simulink model "top_model_24a"  (R2024a)
settings: Solver=VariableStepAuto  StartTime=0.0  StopTime=90  RelTol=1e-3  EnableMultiTasking=on
values from neighbouring files (symbols this model uses):
  target = waypoints(idx, :)'    [waypointFollower - Copy.m]    (also in waypointFollower.m)
undefined symbols (not defined in the file or in its folder): controller, gray, vehicle, X, Y, Z
libraries: sm_lib x13, nesl_utility x6, simulink x5, slpidlib x2, robotmobilelib x1
(part 1 of 2)
settings Model: Creator=The MathWorks, Inc.  LastModifiedBy=s1706516
settings SolverCC: AlgebraicLoopSolver=TrustRegion
settings DataIOCC: LimitDataPoints=on  ReturnWorkspaceOutputs=off
settings OptimizationCC: LifeSpan=inf
settings DebuggingCC: UnconnectedInputMsg=warning  UnconnectedOutputMsg=warning  UnconnectedLineMsg=warning  AllowSymbolicDim=off  SFUnexpectedBacktrackingDiag=warning  SFNoUnconditionalDefaultTransitionDiag=warning  SFExecutionAtInitializationDiag=none  ArithmeticOperatorsInVariantConditions=warning
settings ModelReferenceCC: EnableRefExpFcnMdlSchedulingChecks=on  PropagateSignalLabelsOutOfModel=off
settings SFSimCC: SimUseLocalCustomCode=off  CustomCodeUndefinedFunction=UseInterfaceOnly
settings RTWCC: RTWUseLocalCustomCode=off  GPUComputeCapability=3.5
settings CodeAppCC: StateflowObjectComments=on
settings GRTTargetCC: TargetLangStandard=C89/C90 (ANSI)
settings ConfigComp: CovMetricSettings=dw  CovSaveCumulativeToWorkspaceVar=on  CovSaveSingleToWorkspaceVar=on  CovExternalEMLEnable=off
settings ExplorerConfigSet: InternalSimMechanicsExplorerSettings="<ExplorerConfiguration><canonicalview>default</canonicalview><AnimationSetting><BasePlaybackSpeed>1.0</BasePlaybackSpeed><PlaybackSpeedFactor>1.0</PlaybackSpeedFactor></AnimationSetting><TilePanel><TileInfo><Tiles Columns=\"1\" Count=\"1\" Rows=\"1\"><Column Weight=\"1\"/><Row Weight=\"1\"/><Tile Height=\"1\" Width=\"1\" X=\"0\" Y=\"0\"/></Tiles></TileInfo><SceneInfo><SceneViewer><BGColor><R>0.60000002384185791</R><G>0.60000002384185791</G><B>0.60000002384185791</B></BGColor><Camera><DoPerspective>off</DoPerspective><Position><X>8.17861551168531875</X><Y>-8.17861559442319219</Y><Z>8.17861528352223388</Z></Position><Center><X>9.49663426935732896e-08</X><Y>-1.77704216256942048e-07</Y><Z>-1.33196743078566375e-07</Z></Center><Up><X>-0.408248290463863073</X><Y>0.408248290463863073</Y><Z>0.816496580927726145</Z></Up><ViewLimDist>1</ViewLimDist><YLim>8.40991459846496525</YLim><XLim>17.077552386237727</XLim></Camera></SceneViewer></SceneInfo></TilePanel><MechEditorPanel><Cameras/><GfxPanelCameraMap/><VideoCreator><PlaybackSpeedRatio>1.0</PlaybackSpeedRatio><FrameRate>30</FrameRate><VideoFormat>Motion JPEG AVI</VideoFormat><FrameSize>auto</FrameSize></VideoCreator></MechEditorPanel></ExplorerConfiguration>"

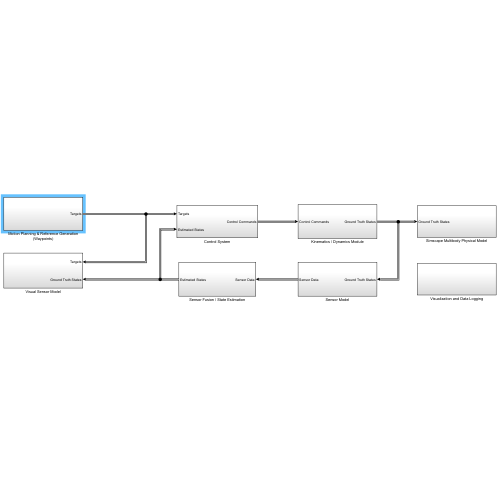
[thumbnail: Simulink's stored preview of the top-level diagram]
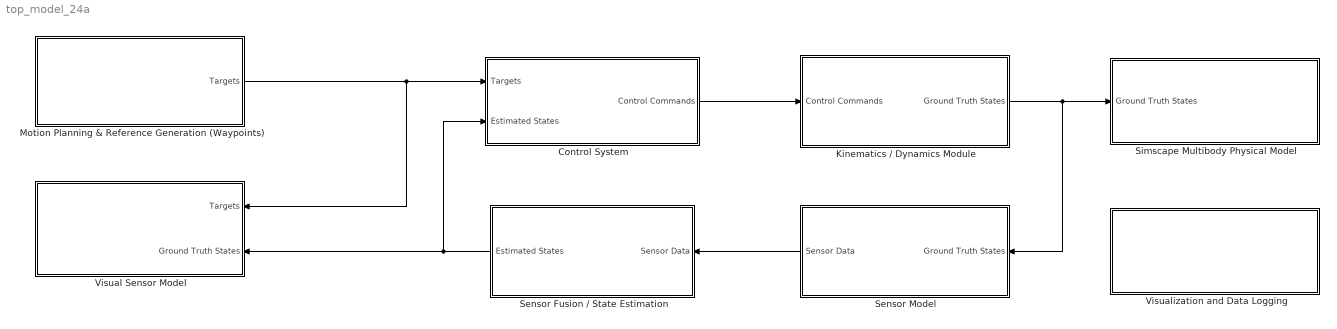
== system top_model_24a ==
  Control System : Subsystem
  Kinematics / Dynamics Module : Subsystem
  Motion Planning & Reference Generation (Waypoints) : Subsystem
  Sensor Fusion / State Estimation : Subsystem
  Sensor Model : Subsystem
  Simscape Multibody Physical Model : Subsystem
  Visual Sensor Model : Subsystem
  Visualization and Data Logging : Subsystem
  wires:
  Sensor Model/1(Sensor Data) -> Sensor Fusion / State Estimation/1(Sensor Data)
  Sensor Fusion / State Estimation/1(Estimated States) -> Visual Sensor Model/2(Ground Truth States), Control System/2(Estimated States)
  Control System/1(Control Commands) -> Kinematics / Dynamics Module/1(Control Commands)
  Kinematics / Dynamics Module/1(Ground Truth States) -> Sensor Model/1(Ground Truth States), Simscape Multibody Physical Model/1(Ground Truth States)
  Motion Planning & Reference Generation (Waypoints)/1(Targets) -> Visual Sensor Model/1(Targets), Control System/1(Targets)

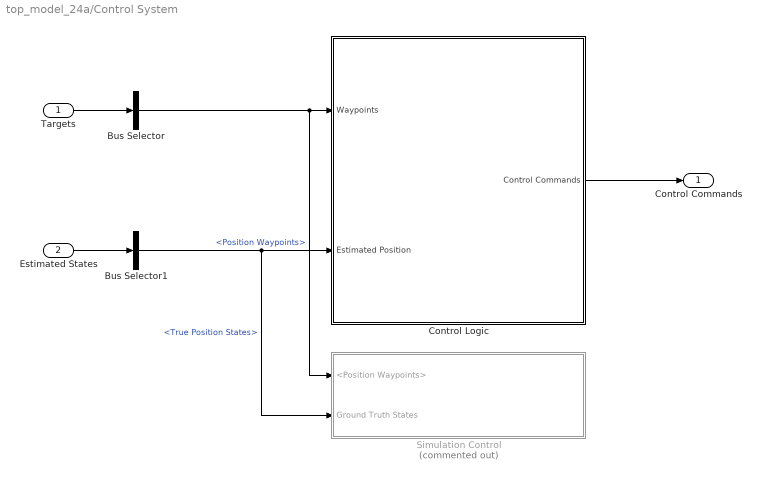
== system top_model_24a/Control System ==
  Targets : Inport
  Estimated States : Inport  Port=2
  Bus Selector : BusSelector  OutputSignals=Position Waypoints
  Bus Selector1 : BusSelector  OutputSignals=True Position States
  Control Logic : Subsystem
  Simulation Control : Subsystem  Commented=on
  Control Commands : Outport
  wires:
  Estimated States/1 -> Bus Selector1/1
  Bus Selector/1 -> Simulation Control/1(<Position Waypoints>), Control Logic/1(Waypoints)  "<Position Waypoints>"
  Targets/1 -> Bus Selector/1
  Control Logic/1(Control Commands) -> Control Commands/1
  Bus Selector1/1 -> Simulation Control/2(Ground Truth States), Control Logic/2(Estimated Position)  "<True Position States>"

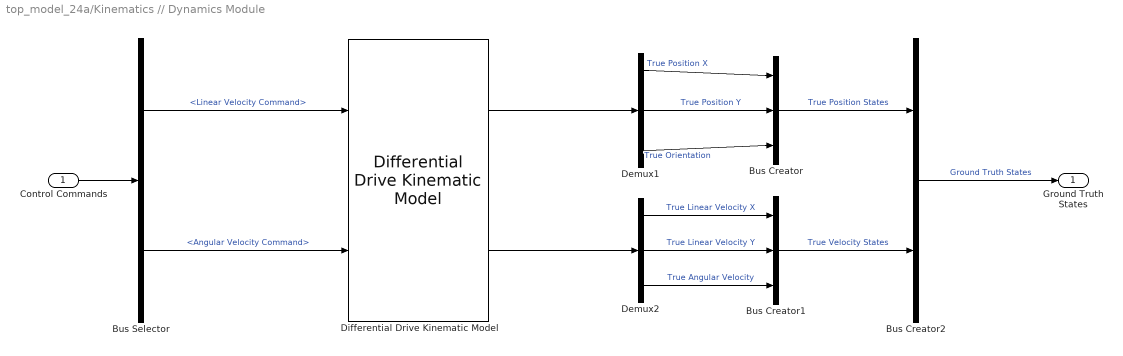
== system top_model_24a/Kinematics // Dynamics Module ==
  Control Commands : Inport
  Bus Creator : BusCreator  Inputs=3
  Bus Creator1 : BusCreator  Inputs=3
  Bus Creator2 : BusCreator  Inputs=2
  Bus Selector : BusSelector  OutputSignals=Linear Velocity Command,Angular Velocity Command
  Demux1 : Demux  Outputs=3
  Demux2 : Demux  Outputs=3
  Differential Drive Kinematic Model : robotmobilelib/Differential Drive Kinematic Model  VehicleInputs=Vehicle Speed & Heading Angular Velocity  WheelRadius=vehicle.wheel.radius  WheelSpeedRange=[-inf inf]  TrackWidth=vehicle.wheel.width  InitialState=init.vehicle.state  SimulateUsing=Interpreted execution
  Ground Truth States : Outport
  wires:
  Bus Selector/1 -> Differential Drive Kinematic Model/1  "<Linear Velocity Command>"
  Bus Selector/2 -> Differential Drive Kinematic Model/2  "<Angular Velocity Command>"
  Control Commands/1 -> Bus Selector/1
  Differential Drive Kinematic Model/1 -> Demux1/1
  Demux1/2 -> Bus Creator/2  "True Position Y"
  Demux1/1 -> Bus Creator/1  "True Position X"
  Demux1/3 -> Bus Creator/3  "True Orientation"
  Differential Drive Kinematic Model/2 -> Demux2/1
  Demux2/1 -> Bus Creator1/1  "True Linear Velocity X"
  Demux2/3 -> Bus Creator1/3  "True Angular Velocity"
  Demux2/2 -> Bus Creator1/2  "True Linear Velocity Y"
  Bus Creator/1 -> Bus Creator2/1  "True Position States"
  Bus Creator1/1 -> Bus Creator2/2  "True Velocity States"
  Bus Creator2/1 -> Ground Truth States/1  "Ground Truth States"

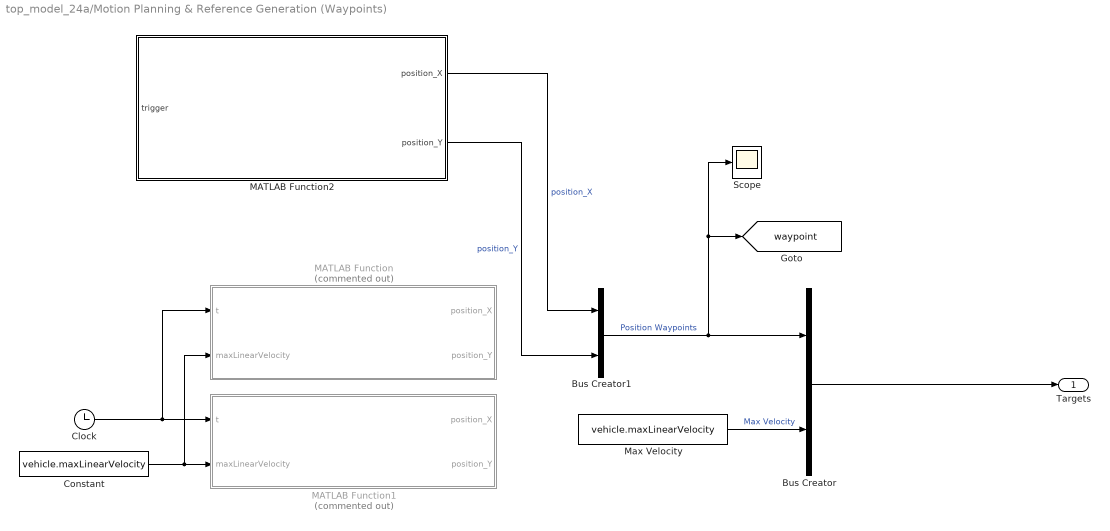
== system top_model_24a/Motion Planning & Reference Generation (Waypoints) ==
  Bus Creator : BusCreator  Inputs=2
  Bus Creator1 : BusCreator  Inputs=2
  Clock : Clock
  Constant : Constant  Value=vehicle.maxLinearVelocity
  MATLAB Function : MATLAB Function  Commented=on  TreatAsAtomicUnit=on
  MATLAB Function1 : MATLAB Function  Commented=on  TreatAsAtomicUnit=on
  MATLAB Function2 : MATLAB Function  TreatAsAtomicUnit=on
  Max Velocity : Constant  Value=vehicle.maxLinearVelocity
  Scope : Scope
  Targets : Outport
  tag scope: waypoint=global
  wires:
  Max Velocity/1 -> Bus Creator/2  "Max Velocity"
  Bus Creator/1 -> Targets/1
  Bus Creator1/1 -> Bus Creator/1, [waypoint], Scope/1  "Position Waypoints"
  Constant/1 -> MATLAB Function/2(maxLinearVelocity), MATLAB Function1/2(maxLinearVelocity)
  Clock/1 -> MATLAB Function/1(t), MATLAB Function1/1(t)
  MATLAB Function2/1(position_X) -> Bus Creator1/1  "position_X"
  MATLAB Function2/2(position_Y) -> Bus Creator1/2  "position_Y"

== system top_model_24a/Sensor Fusion // State Estimation ==
  Sensor Data : Inport
  Bus Creator : BusCreator  Inputs=2
  Bus Selector : BusSelector  OutputSignals=True Position States,True Velocity States
  Sensor Fusion : Subsystem
  Estimated States : Outport
  wires:
  Sensor Data/1 -> Bus Selector/1  "Sensor Data"
  Bus Creator/1 -> Estimated States/1  "Estimated States"
  Bus Selector/1 -> Sensor Fusion/1(In1)  "<True Position States>"
  Bus Selector/2 -> Sensor Fusion/2(In2)  "<True Velocity States>"
  Sensor Fusion/1(Out1) -> Bus Creator/1
  Sensor Fusion/2(Out2) -> Bus Creator/2

== system top_model_24a/Sensor Model ==
  Ground Truth States : Inport
  Sensors : Subsystem
  Switch : simulink/Signal Routing/Manual Variant Source  NumChoices=2  LabelModeActiveChoice=V_1
  True Feedthrough : Subsystem
  Sensor Data : Outport
  wires:
  Switch/1 -> Sensor Data/1
  Ground Truth States/1 -> True Feedthrough/1(Ground Truth States), Sensors/1(Ground Truth States)
  Sensors/1(Simulated Raw Sensor Data) -> Switch/1  "Sensor Data"
  True Feedthrough/1(True Feedthrough Sensor Data) -> Switch/2  "Sensor Data"

== system top_model_24a/Simscape Multibody Physical Model ==
  Ground Truth States : Inport
  Bus Selector : BusSelector  OutputSignals=True Position States
  Simscape Model : Subsystem
  wires:
  Ground Truth States/1 -> Bus Selector/1
  Bus Selector/1 -> Simscape Model/1(True Position States)  "<True Position States>"

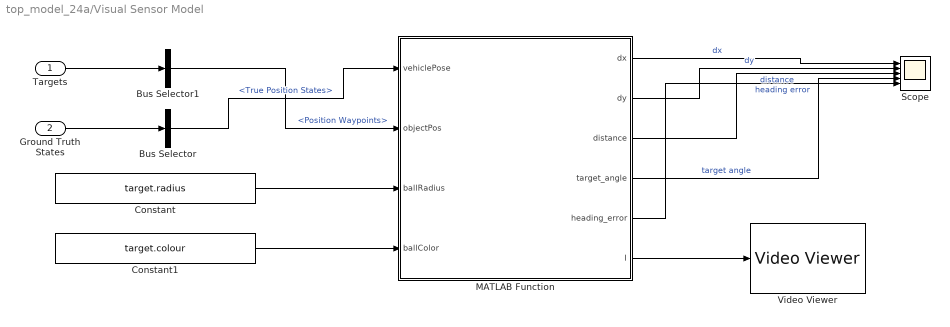
== system top_model_24a/Visual Sensor Model ==
  Targets : Inport
  Ground Truth States : Inport  Port=2
  Bus Selector : BusSelector  OutputSignals=True Position States
  Bus Selector1 : BusSelector  OutputSignals=Position Waypoints
  Constant : Constant  Value=target.radius
  Constant1 : Constant  Value=target.colour
  MATLAB Function : MATLAB Function  TreatAsAtomicUnit=on
  Scope : Scope  NumInputPorts=5
  Video Viewer : VideoViewer  colormapValue=gray(256)  FigPos=[830 505 439 384]
  wires:
  Ground Truth States/1 -> Bus Selector/1
  Bus Selector/1 -> MATLAB Function/1(vehiclePose)  "<True Position States>"
  Targets/1 -> Bus Selector1/1
  Bus Selector1/1 -> MATLAB Function/2(objectPos)  "<Position Waypoints>"
  MATLAB Function/6(I) -> Video Viewer/1
  Constant/1 -> MATLAB Function/3(ballRadius)
  Constant1/1 -> MATLAB Function/4(ballColor)
  MATLAB Function/1(dx) -> Scope/1  "dx"
  MATLAB Function/2(dy) -> Scope/2  "dy"
  MATLAB Function/4(target_angle) -> Scope/4  "target angle"
  MATLAB Function/5(heading_error) -> Scope/5  "heading error"
  MATLAB Function/3(distance) -> Scope/3  "distance"

== system top_model_24a/Visualization and Data Logging ==

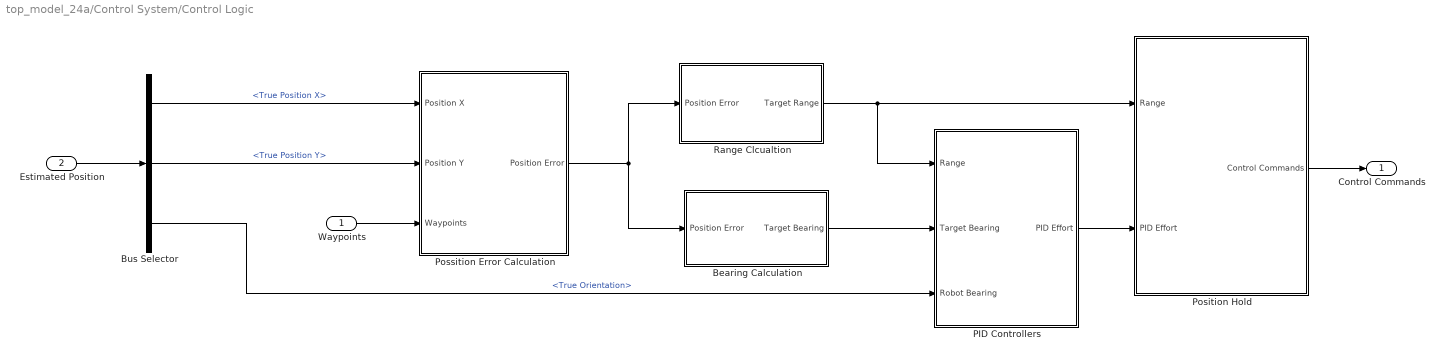
== system top_model_24a/Control System/Control Logic ==
  Waypoints : Inport
  Estimated Position : Inport  Port=2
  Bearing Calculation : Subsystem
  Bus Selector : BusSelector  OutputSignals=True Position X,True Position Y,True Orientation
  PID Controllers : Subsystem
  Position Hold : Subsystem
  Possition Error Calculation : Subsystem
  Range Clcualtion : Subsystem
  Control Commands : Outport
  wires:
  Waypoints/1 -> Possition Error Calculation/3(Waypoints)
  Estimated Position/1 -> Bus Selector/1
  Bus Selector/3 -> PID Controllers/3(Robot Bearing)  "<True Orientation>"
  Position Hold/1(Control Commands) -> Control Commands/1
  Bearing Calculation/1(Target Bearing) -> PID Controllers/2(Target Bearing)
  Possition Error Calculation/1(Position Error) -> Range Clcualtion/1(Position Error), Bearing Calculation/1(Position Error)
  Bus Selector/1 -> Possition Error Calculation/1(Position X)  "<True Position X>"
  Bus Selector/2 -> Possition Error Calculation/2(Position Y)  "<True Position Y>"
  Range Clcualtion/1(Target Range) -> PID Controllers/1(Range), Position Hold/1(Range)
  PID Controllers/1(PID Effort) -> Position Hold/2(PID Effort)

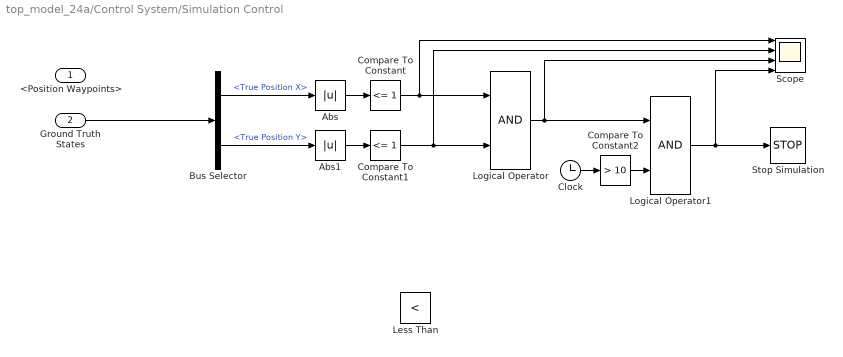
== system top_model_24a/Control System/Simulation Control ==
  <Position Waypoints> : Inport
  Ground Truth States : Inport  Port=2
  Abs : Abs  SaturateOnIntegerOverflow=off
  Abs1 : Abs  SaturateOnIntegerOverflow=off
  Bus Selector : BusSelector  OutputSignals=True Position X,True Position Y
  Clock : Clock
  Compare To Constant : simulink/Logic and Bit Operations/Compare To Constant  relop=<=  const=1  OutDataTypeStr=boolean
  Compare To Constant1 : simulink/Logic and Bit Operations/Compare To Constant  relop=<=  const=1  OutDataTypeStr=boolean
  Compare To Constant2 : simulink/Logic and Bit Operations/Compare To Constant  relop=>  const=10  OutDataTypeStr=boolean
  Less Than : RelationalOperator  Operator=<  OutDataTypeStr=boolean  RndMeth=Simplest  InputSameDT=off
  Logical Operator : Logic  AllPortsSameDT=off  OutDataTypeStr=boolean
  Logical Operator1 : Logic  AllPortsSameDT=off  OutDataTypeStr=boolean
  Scope : Scope  NumInputPorts=4
  Stop Simulation : Stop
  wires:
  Ground Truth States/1 -> Bus Selector/1
  Bus Selector/1 -> Abs/1  "<True Position X>"
  Bus Selector/2 -> Abs1/1  "<True Position Y>"
  Compare To Constant/1 -> Logical Operator/1, Scope/1
  Compare To Constant1/1 -> Logical Operator/2, Scope/2
  Logical Operator/1 -> Logical Operator1/1, Scope/3
  Abs/1 -> Compare To Constant/1
  Abs1/1 -> Compare To Constant1/1
  Compare To Constant2/1 -> Logical Operator1/2
  Clock/1 -> Compare To Constant2/1
  Logical Operator1/1 -> Stop Simulation/1, Scope/4

== system top_model_24a/Sensor Fusion // State Estimation/Sensor Fusion ==
  In1 : Inport
  In2 : Inport  Port=2
  Out1 : Outport
  Out2 : Outport  Port=2
  wires:
  In1/1 -> Out1/1
  In2/1 -> Out2/1

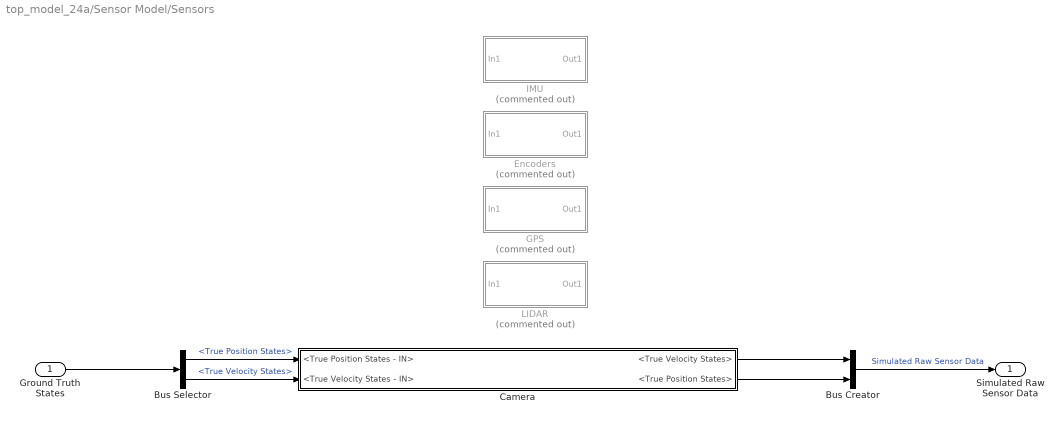
== system top_model_24a/Sensor Model/Sensors ==
  Ground Truth States : Inport
  Bus Creator : BusCreator  Inputs=2
  Bus Selector : BusSelector  OutputSignals=True Position States,True Velocity States
  Camera : Subsystem
  Encoders : Subsystem  Commented=on
  GPS : Subsystem  Commented=on
  IMU : Subsystem  Commented=on
  LIDAR : Subsystem  Commented=on
  Simulated Raw Sensor Data : Outport
  wires:
  Ground Truth States/1 -> Bus Selector/1
  Bus Creator/1 -> Simulated Raw Sensor Data/1  "Simulated Raw Sensor Data"
  Camera/2(<True Position States>) -> Bus Creator/2
  Bus Selector/2 -> Camera/2(<True Velocity States - IN>)  "<True Velocity States>"
  Bus Selector/1 -> Camera/1(<True Position States - IN>)  "<True Position States>"
  Camera/1(<True Velocity States>) -> Bus Creator/1

== system top_model_24a/Sensor Model/True Feedthrough ==
  Ground Truth States : Inport
  Bus Creator : BusCreator  Inputs=2
  Bus Selector : BusSelector  OutputSignals=True Position States,True Velocity States
  True Feedthrough Sensor Data : Outport
  wires:
  Bus Creator/1 -> True Feedthrough Sensor Data/1  "True Feedthrough Sensor Data"
  Ground Truth States/1 -> Bus Selector/1
  Bus Selector/1 -> Bus Creator/1  "<True Position States>"
  Bus Selector/2 -> Bus Creator/2  "<True Velocity States>"

== system top_model_24a/Simscape Multibody Physical Model/Simscape Model ==
  True Position States : Inport
  Vehicle Base : Subsystem
  World and Solver : Subsystem
  wires:
  True Position States/1 -> Vehicle Base/1(True Position States)
  connections:
  World and Solver/RConn1 -- Vehicle Base/LConn1

== system top_model_24a/Control System/Control Logic/Bearing Calculation ==
  Position Error : Inport
  Atan1 : Trigonometry  Operator=atan2
  Demux1 : Demux  Outputs=2
  Target Bearing : Outport
  wires:
  Demux1/2 -> Atan1/1
  Demux1/1 -> Atan1/2
  Atan1/1 -> Target Bearing/1
  Position Error/1 -> Demux1/1

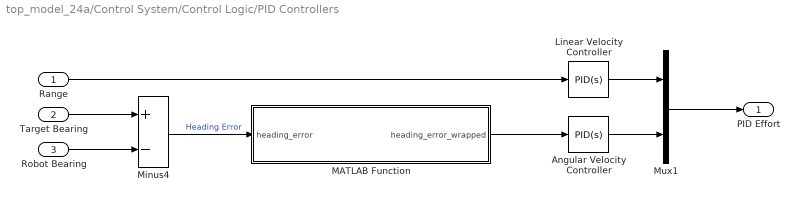
== system top_model_24a/Control System/Control Logic/PID Controllers ==
  Range : Inport
  Target Bearing : Inport  Port=2
  Robot Bearing : Inport  Port=3
  Angular Velocity Controller : slpidlib/PID Controller  Controller=PID  Form=Parallel  TimeDomain=Continuous-time  UseExternalTs=off  SampleTime=-1  IntegratorMethod=Forward Euler  FilterMethod=Forward Euler  ControllerParametersSource=internal  P=1  I=0  UseKiTs=off  D=0.1  UseExternalDerivativeSource=off  N=1  UseFilter=on  TunerSelectOption=Transfer Function Based (PID Tuner App)  InitialConditionSource=internal  InitialConditionForIntegrator=0  InitialConditionForFilter=0  DifferentiatorICPrevScaledInput=0  ExternalReset=none  TrackingMode=off  Kt=1  LimitOutput=off  SatLimitsSource=internal  UpperSaturationLimit=inf  LowerSaturationLimit=-inf  LinearizeAsGain=on  AntiWindupMode=none  Kb=1  LimitIntegrator=off  UpperIntegratorSaturationLimit=inf  LowerIntegratorSaturationLimit=-inf  POutMin=[]  POutMax=[]  IOutMin=[]  IOutMax=[]  DOutMin=[]  DOutMax=[]  NOutMin=[]  NOutMax=[]  SumOutMin=[]  SumOutMax=[]  SaturationOutMin=[]  SaturationOutMax=[]  PParamMin=[]  PParamMax=[]  IParamMin=[]  IParamMax=[]  DParamMin=[]  DParamMax=[]  NParamMin=[]  NParamMax=[]  KbParamMin=[]  KbParamMax=[]  KtParamMin=[]  KtParamMax=[]  KbOutMin=[]  KbOutMax=[]  KtOutMin=[]  KtOutMax=[]  IntegratorOutMin=[]  IntegratorOutMax=[]  FilterOutMin=[]  FilterOutMax=[]  SumI1OutMin=[]  SumI1OutMax=[]  SumI2OutMin=[]  SumI2OutMax=[]  SumI3OutMin=[]  SumI3OutMax=[]  SumI4OutMin=[]  SumI4OutMax=[]  SumDOutMin=[]  SumDOutMax=[]  DifferentiatorOutMin=[]  DifferentiatorOutMax=[]  FilterDiffOutCoefMin=[]  FilterDiffOutCoefMax=[]  ReciprocalOutMin=[]  ReciprocalOutMax=[]  SumDenOutMin=[]  SumDenOutMax=[]  SumNumOutMin=[]  SumNumOutMax=[]  DivideOutMin=[]  DivideOutMax=[]  UdiffTsProdOutMin=[]  UdiffTsProdOutMax=[]  NTsProdOutMin=[]  NTsProdOutMax=[]  UintegralTsProdOutMin=[]  UintegralTsProdOutMax=[]  UngainTsProdOutMin=[]  UngainTsProdOutMax=[]  ClampingZeroOutDataTypeStr=Inherit: Inherit via back propagation  ClampingZeroOutMin=[]  ClampingZeroOutMax=[]  FilterDenConstantOutDataTypeStr=Inherit: Inherit via back propagation  FilterDenConstantOutMin=[]  FilterDenConstantOutMax=[]  PCopyOutDataTypeStr=Inherit: Inherit via back propagation  PCopyOutMin=[]  PCopyOutMax=[]  NCopyOutDataTypeStr=Inherit: Inherit via back propagation  NCopyOutMin=[]  NCopyOutMax=[]  IntegratorContinuousStateAttributes=''  IntegratorStateMustResolveToSignalObject=off  IntegratorRTWStateStorageClass=Auto  FilterContinuousStateAttributes=''  FilterStateMustResolveToSignalObject=off  FilterRTWStateStorageClass=Auto  ParallelPVariant=InternalParameters  IdealPVariant=Disabled  IVariant=InternalParameters  DVariant=InternalParameters  IntegratorVariant=Continuous  SatVariant=Disabled  AWVariant=Passthrough  PCopyVariant=Disabled  TRVariant=Disabled  FdbkBlocksVariant=Forward  IdealPFdbkVariant=Disabled  SatFdbkVariant=Disabled  DerivativeFilterVariant=ContFilter  NVariant=InternalParameters  NCopyVariant=Disabled  FilterICVariant=InternalICsFilter  IntegratorICVariant=InternalICs  ExternalResetVariant=Disabled  TRSumVariant=Passthrough  SumFdbkVariant=Disabled  SumVariant=Sum_PID  TsampFilterVariant=InternalTs  TsampNgainVariant=Passthrough  TsampIntegralVariant=Disabled_SignalSpec  ExternalSaturationOutDataTypeStr=Inherit: Same as second input  DerivativeSourceVariant=ErrorSignal
  Linear Velocity Controller : slpidlib/PID Controller  Controller=PID  Form=Parallel  TimeDomain=Continuous-time  UseExternalTs=off  SampleTime=-1  IntegratorMethod=Forward Euler  FilterMethod=Forward Euler  ControllerParametersSource=internal  P=1  I=0  UseKiTs=off  D=0.1  UseExternalDerivativeSource=off  N=1  UseFilter=on  TunerSelectOption=Transfer Function Based (PID Tuner App)  InitialConditionSource=internal  InitialConditionForIntegrator=0  InitialConditionForFilter=0  DifferentiatorICPrevScaledInput=0  ExternalReset=none  TrackingMode=off  Kt=1  LimitOutput=off  SatLimitsSource=internal  UpperSaturationLimit=inf  LowerSaturationLimit=-inf  LinearizeAsGain=on  AntiWindupMode=none  Kb=1  LimitIntegrator=off  UpperIntegratorSaturationLimit=inf  LowerIntegratorSaturationLimit=-inf  POutMin=[]  POutMax=[]  IOutMin=[]  IOutMax=[]  DOutMin=[]  DOutMax=[]  NOutMin=[]  NOutMax=[]  SumOutMin=[]  SumOutMax=[]  SaturationOutMin=[]  SaturationOutMax=[]  PParamMin=[]  PParamMax=[]  IParamMin=[]  IParamMax=[]  DParamMin=[]  DParamMax=[]  NParamMin=[]  NParamMax=[]  KbParamMin=[]  KbParamMax=[]  KtParamMin=[]  KtParamMax=[]  KbOutMin=[]  KbOutMax=[]  KtOutMin=[]  KtOutMax=[]  IntegratorOutMin=[]  IntegratorOutMax=[]  FilterOutMin=[]  FilterOutMax=[]  SumI1OutMin=[]  SumI1OutMax=[]  SumI2OutMin=[]  SumI2OutMax=[]  SumI3OutMin=[]  SumI3OutMax=[]  SumI4OutMin=[]  SumI4OutMax=[]  SumDOutMin=[]  SumDOutMax=[]  DifferentiatorOutMin=[]  DifferentiatorOutMax=[]  FilterDiffOutCoefMin=[]  FilterDiffOutCoefMax=[]  ReciprocalOutMin=[]  ReciprocalOutMax=[]  SumDenOutMin=[]  SumDenOutMax=[]  SumNumOutMin=[]  SumNumOutMax=[]  DivideOutMin=[]  DivideOutMax=[]  UdiffTsProdOutMin=[]  UdiffTsProdOutMax=[]  NTsProdOutMin=[]  NTsProdOutMax=[]  UintegralTsProdOutMin=[]  UintegralTsProdOutMax=[]  UngainTsProdOutMin=[]  UngainTsProdOutMax=[]  ClampingZeroOutDataTypeStr=Inherit: Inherit via back propagation  ClampingZeroOutMin=[]  ClampingZeroOutMax=[]  FilterDenConstantOutDataTypeStr=Inherit: Inherit via back propagation  FilterDenConstantOutMin=[]  FilterDenConstantOutMax=[]  PCopyOutDataTypeStr=Inherit: Inherit via back propagation  PCopyOutMin=[]  PCopyOutMax=[]  NCopyOutDataTypeStr=Inherit: Inherit via back propagation  NCopyOutMin=[]  NCopyOutMax=[]  IntegratorContinuousStateAttributes=''  IntegratorStateMustResolveToSignalObject=off  IntegratorRTWStateStorageClass=Auto  FilterContinuousStateAttributes=''  FilterStateMustResolveToSignalObject=off  FilterRTWStateStorageClass=Auto  ParallelPVariant=InternalParameters  IdealPVariant=Disabled  IVariant=InternalParameters  DVariant=InternalParameters  IntegratorVariant=Continuous  SatVariant=Disabled  AWVariant=Passthrough  PCopyVariant=Disabled  TRVariant=Disabled  FdbkBlocksVariant=Forward  IdealPFdbkVariant=Disabled  SatFdbkVariant=Disabled  DerivativeFilterVariant=ContFilter  NVariant=InternalParameters  NCopyVariant=Disabled  FilterICVariant=InternalICsFilter  IntegratorICVariant=InternalICs  ExternalResetVariant=Disabled  TRSumVariant=Passthrough  SumFdbkVariant=Disabled  SumVariant=Sum_PID  TsampFilterVariant=InternalTs  TsampNgainVariant=Passthrough  TsampIntegralVariant=Disabled_SignalSpec  ExternalSaturationOutDataTypeStr=Inherit: Same as second input  DerivativeSourceVariant=ErrorSignal
  MATLAB Function : MATLAB Function  TreatAsAtomicUnit=on
  Minus4 : Sum  Inputs=+-
  Mux1 : Mux  Inputs=2
  PID Effort : Outport
  wires:
  Linear Velocity Controller/1 -> Mux1/1
  Angular Velocity Controller/1 -> Mux1/2
  Minus4/1 -> MATLAB Function/1(heading_error)  "Heading Error"
  Range/1 -> Linear Velocity Controller/1
  Mux1/1 -> PID Effort/1
  Target Bearing/1 -> Minus4/1
  Robot Bearing/1 -> Minus4/2
  MATLAB Function/1(heading_error_wrapped) -> Angular Velocity Controller/1

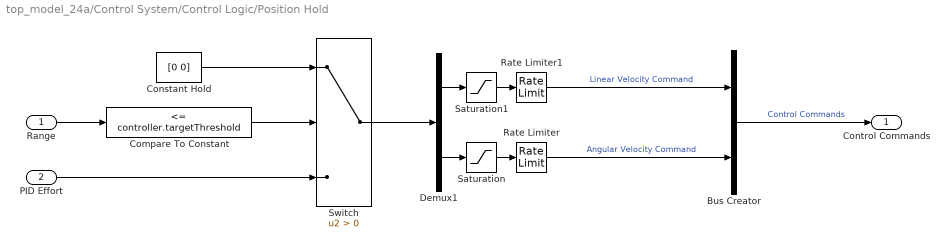
== system top_model_24a/Control System/Control Logic/Position Hold ==
  Range : Inport
  PID Effort : Inport  Port=2
  Bus Creator : BusCreator  Inputs=2
  Compare To Constant : simulink/Logic and Bit Operations/Compare To Constant  relop=<=  const=controller.targetThreshold  OutDataTypeStr=boolean
  Constant Hold : Constant  Value=[0 0]
  Demux1 : Demux  Outputs=2
  Rate Limiter : RateLimiter  RisingSlewLimit=vehicle.maxAngularAcceleration  FallingSlewLimit=-vehicle.maxAngularAcceleration  SampleTimeMode=inherited
  Rate Limiter1 : RateLimiter  RisingSlewLimit=vehicle.maxLinearAcceleration  FallingSlewLimit=-vehicle.maxLinearAcceleration  SampleTimeMode=inherited
  Saturation : Saturate  UpperLimit=vehicle.maxAngularVelocity  LowerLimit=-vehicle.maxAngularVelocity
  Saturation1 : Saturate  UpperLimit=vehicle.maxLinearVelocity  LowerLimit=-vehicle.maxLinearVelocity
  Switch : Switch  Criteria=u2 > Threshold  SaturateOnIntegerOverflow=off  InputSameDT=off
  Control Commands : Outport
  wires:
  PID Effort/1 -> Switch/3
  Range/1 -> Compare To Constant/1
  Constant Hold/1 -> Switch/1
  Switch/1 -> Demux1/1
  Rate Limiter1/1 -> Bus Creator/1  "Linear Velocity Command"
  Rate Limiter/1 -> Bus Creator/2  "Angular Velocity Command"
  Bus Creator/1 -> Control Commands/1  "Control Commands"
  Saturation/1 -> Rate Limiter/1
  Saturation1/1 -> Rate Limiter1/1
  Demux1/1 -> Saturation1/1
  Demux1/2 -> Saturation/1
  Compare To Constant/1 -> Switch/2

== system top_model_24a/Control System/Control Logic/Possition Error Calculation ==
  Position X : Inport
  Position Y : Inport  Port=2
  Waypoints : Inport  Port=3
  Minus3 : Sum  Inputs=+-
  Mux : Mux  Inputs=2
  Position Error : Outport
  wires:
  Mux/1 -> Minus3/2
  Position Y/1 -> Mux/2
  Waypoints/1 -> Minus3/1
  Minus3/1 -> Position Error/1
  Position X/1 -> Mux/1

== system top_model_24a/Control System/Control Logic/Range Clcualtion ==
  Position Error : Inport
  Square Root1 : Sqrt
  Square2 : Math  Operator=square
  Sum of Elements : Sum  Inputs=+
  Target Range : Outport
  wires:
  Sum of Elements/1 -> Square Root1/1
  Square2/1 -> Sum of Elements/1
  Square Root1/1 -> Target Range/1  "Range"
  Position Error/1 -> Square2/1

== system top_model_24a/Sensor Model/Sensors/Camera ==
  <True Position States - IN> : Inport
  <True Velocity States - IN> : Inport  Port=2
  MATLAB Function : MATLAB Function  TreatAsAtomicUnit=on
  Video Viewer : VideoViewer  Commented=on  colormapValue=gray(256)  FigPos=[2458 385 418 304]
  <True Velocity States> : Outport
  <True Position States> : Outport  Port=2
  wires:
  <True Position States - IN>/1 -> <True Position States>/1, MATLAB Function/1(pose)
  <True Velocity States - IN>/1 -> <True Velocity States>/1
  MATLAB Function/1(I) -> Video Viewer/1

== system top_model_24a/Sensor Model/Sensors/Encoders ==
  In1 : Inport
  Out1 : Outport
  wires:
  In1/1 -> Out1/1

== system top_model_24a/Sensor Model/Sensors/GPS ==
  In1 : Inport
  Out1 : Outport
  wires:
  In1/1 -> Out1/1

== system top_model_24a/Sensor Model/Sensors/IMU ==
  In1 : Inport
  Out1 : Outport
  wires:
  In1/1 -> Out1/1

== system top_model_24a/Sensor Model/Sensors/LIDAR ==
  In1 : Inport
  Out1 : Outport
  wires:
  In1/1 -> Out1/1

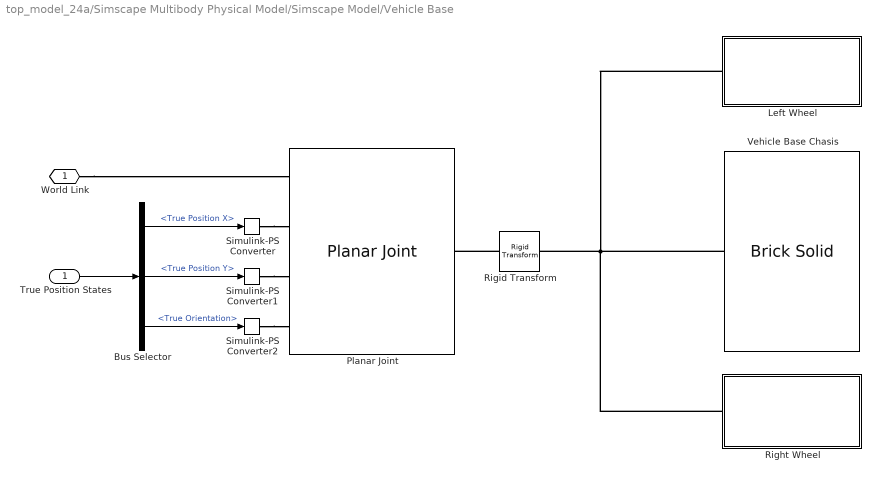
== system top_model_24a/Simscape Multibody Physical Model/Simscape Model/Vehicle Base ==
  True Position States : Inport
  Bus Selector : BusSelector  OutputSignals=True Position X,True Position Y,True Orientation
  Left Wheel : Subsystem
  Planar Joint : sm_lib/Joints/Planar Joint  JointMode=Normal  CompositeWrenchDir=FollowerOnBase  CompositeWrenchFrame=BaseFrame  SenseConstraintForce=off  SenseConstraintTorque=off  SenseTotalForce=off  SenseTotalTorque=off  PxPositionTargetSpecify=off  PxPositionTargetPriority=High  PxPositionTargetValue=0  PxPositionTargetValueUnits=m  PxVelocityTargetSpecify=off  PxVelocityTargetPriority=High  PxVelocityTargetValue=0  PxVelocityTargetValueUnits=m/s  PxEquilibriumPosition=0  PxEquilibriumPositionUnits=m  PxSpringStiffness=0  PxSpringStiffnessUnits=N/m  PxDampingCoefficient=0  PxDampingCoefficientUnits=N/(m/s)  PxLowerLimitSpecify=off  PxLowerLimitBound=-1  PxLowerLimitBoundUnits=m  PxLowerLimitStiffness=1e6  PxLowerLimitStiffnessUnits=N/m  PxLowerLimitDamping=1e3  PxLowerLimitDampingUnits=N/(m/s)  PxLowerLimitTransitionRegionWidth=1e-4  PxLowerLimitTransitionRegionWidthUnits=m  PxUpperLimitSpecify=off  PxUpperLimitBound=1  PxUpperLimitBoundUnits=m  PxUpperLimitStiffness=1e6  PxUpperLimitStiffnessUnits=N/m  PxUpperLimitDamping=1e3  PxUpperLimitDampingUnits=N/(m/s)  PxUpperLimitTransitionRegionWidth=1e-4  PxUpperLimitTransitionRegionWidthUnits=m  PxTorqueActuationMode=ComputedTorque  PxMotionActuationMode=InputMotion  PxSensePosition=off  PxSenseVelocity=off  PxSenseAcceleration=off  PxSenseTorqueForce=off  PxSenseLowerLimitTorqueForce=off  PxSenseUpperLimitTorqueForce=off  PyPositionTargetSpecify=off  PyPositionTargetPriority=High  PyPositionTargetValue=0  PyPositionTargetValueUnits=m  PyVelocityTargetSpecify=off  PyVelocityTargetPriority=High  PyVelocityTargetValue=0  PyVelocityTargetValueUnits=m/s  PyEquilibriumPosition=0  PyEquilibriumPositionUnits=m  PySpringStiffness=0  PySpringStiffnessUnits=N/m  PyDampingCoefficient=0  PyDampingCoefficientUnits=N/(m/s)  PyLowerLimitSpecify=off  PyLowerLimitBound=-1  PyLowerLimitBoundUnits=m  PyLowerLimitStiffness=1e6  PyLowerLimitStiffnessUnits=N/m  PyLowerLimitDamping=1e3  PyLowerLimitDampingUnits=N/(m/s)  PyLowerLimitTransitionRegionWidth=1e-4  PyLowerLimitTransitionRegionWidthUnits=m  PyUpperLimitSpecify=off  PyUpperLimitBound=1  PyUpperLimitBoundUnits=m  PyUpperLimitStiffness=1e6  PyUpperLimitStiffnessUnits=N/m  PyUpperLimitDamping=1e3  PyUpperLimitDampingUnits=N/(m/s)  PyUpperLimitTransitionRegionWidth=1e-4  PyUpperLimitTransitionRegionWidthUnits=m  PyTorqueActuationMode=ComputedTorque  PyMotionActuationMode=InputMotion  PySensePosition=off  PySenseVelocity=off  PySenseAcceleration=off  PySenseTorqueForce=off  PySenseLowerLimitTorqueForce=off  PySenseUpperLimitTorqueForce=off  RzPositionTargetSpecify=off  RzPositionTargetPriority=High  RzPositionTargetValue=0  RzPositionTargetValueUnits=deg  RzVelocityTargetSpecify=off  RzVelocityTargetPriority=High  RzVelocityTargetValue=0  RzVelocityTargetValueUnits=deg/s  RzEquilibriumPosition=0  RzEquilibriumPositionUnits=deg  RzSpringStiffness=0  RzSpringStiffnessUnits=N*m/deg  RzDampingCoefficient=0  RzDampingCoefficientUnits=N*m/(deg/s)  RzLowerLimitSpecify=off  RzLowerLimitBound=-90  RzLowerLimitBoundUnits=deg  RzLowerLimitStiffness=1e4  RzLowerLimitStiffnessUnits=N*m/deg  RzLowerLimitDamping=10  RzLowerLimitDampingUnits=N*m/(deg/s)  RzLowerLimitTransitionRegionWidth=0.1  RzLowerLimitTransitionRegionWidthUnits=deg  RzUpperLimitSpecify=off  RzUpperLimitBound=90  RzUpperLimitBoundUnits=deg  RzUpperLimitStiffness=1e4  RzUpperLimitStiffnessUnits=N*m/deg  RzUpperLimitDamping=10  RzUpperLimitDampingUnits=N*m/(deg/s)  RzUpperLimitTransitionRegionWidth=0.1  RzUpperLimitTransitionRegionWidthUnits=deg  RzTorqueActuationMode=ComputedTorque  RzMotionActuationMode=InputMotion  RzSensePosition=off  RzSenseVelocity=off  RzSenseAcceleration=off  RzSenseTorqueForce=off  RzSenseLowerLimitTorqueForce=off  RzSenseUpperLimitTorqueForce=off
  Right Wheel : Subsystem
  Rigid Transform : sm_lib/Frames and Transforms/Rigid Transform  RotationMethod=None  FollAlignAxisA=+X  BaseAlignAxisA=+X  FollAlignAxisB=+Y  BaseAlignAxisB=+Z  RotationStandardAxis=+Z  RotationAngle=0  RotationAngleUnits=deg  RotationArbitraryAxis=[0 0 1]  RotationSequenceAxes=FollowerAxes  RotationSequence=XYX  RotationSequenceAngles=[0 0 0]  RotationSequenceAnglesUnits=deg  RotationMatrix=[1 0 0;0 1 0;0 0 1]  Quaternion=[1 0 0 0]  TranslationMethod=StandardAxis  TranslationCartesianOffset=[0 0 0]  TranslationCartesianOffsetUnits=m  TranslationStandardAxis=+Z  TranslationStandardOffset=vehicle.baseChasis.groundOffset  TranslationStandardOffsetUnits=m  TranslationROffset=0  TranslationROffsetUnits=m  TranslationThetaOffset=0  TranslationThetaOffsetUnits=deg  TranslationZOffset=0  TranslationZOffsetUnits=m
  Simulink-PS Converter : nesl_utility/Simulink-PS Converter  PhysicalDomain=network_engine_domain  SubClassName=ps_input  LeftPortType=input  RightPortType=output  PseudoPeriodic=off  Frequencies=[]  NoiseDistribution=none  NoiseParameters=[]  Unit=1  AffineConversion=off  FilteringAndDerivatives=filter  SimscapeFilterOrder=2  InputFilterTimeConstant=0.001  UdotUserProvided=0
  Simulink-PS Converter1 : nesl_utility/Simulink-PS Converter  PhysicalDomain=network_engine_domain  SubClassName=ps_input  LeftPortType=input  RightPortType=output  PseudoPeriodic=off  Frequencies=[]  NoiseDistribution=none  NoiseParameters=[]  Unit=1  AffineConversion=off  FilteringAndDerivatives=filter  SimscapeFilterOrder=2  InputFilterTimeConstant=0.001  UdotUserProvided=0
  Simulink-PS Converter2 : nesl_utility/Simulink-PS Converter  PhysicalDomain=network_engine_domain  SubClassName=ps_input  LeftPortType=input  RightPortType=output  PseudoPeriodic=off  Frequencies=[]  NoiseDistribution=none  NoiseParameters=[]  Unit=1  AffineConversion=off  FilteringAndDerivatives=filter  SimscapeFilterOrder=2  InputFilterTimeConstant=0.001  UdotUserProvided=0
  Vehicle Base Chasis : sm_lib/Body Elements/Brick Solid  BrickDimensions=vehicle.baseChasis.dimentions  BrickDimensionsUnits=m  ExportEntireGeometry=off  InertiaType=CalculateFromGeometry  BasedOnType=Mass  Density=1000  DensityUnits=kg/m^3  Mass=vehicle.baseChasis.mass  MassUnits=kg  CenterOfMass=[0 0 0]  CenterOfMassUnits=m  MomentsOfInertia=[1 1 1]  MomentsOfInertiaUnits=kg*m^2  ProductsOfInertia=[0 0 0]  ProductsOfInertiaUnits=kg*m^2  GraphicType=FromGeometry  MarkerShape=Sphere  MarkerSize=10  GraphicVisPropType=SimpleVisualProperties  GraphicDiffuseColor=vehicle.baseChasis.colour  GraphicOpacity=vehicle.baseChasis.opacity  GraphicSpecularColor=[0.5 0.5 0.5 1.0]  GraphicAmbientColor=[0.15 0.15 0.15 1.0]  GraphicEmissiveColor=[0.0 0.0 0.0 1.0]  GraphicShininess=75  DoExposeReferenceFrame=on  SerializedFrames=<Frames/>
  World Link : PMIOPort  Side=Left
  wires:
  Bus Selector/1 -> Simulink-PS Converter/1  "<True Position X>"
  Bus Selector/2 -> Simulink-PS Converter1/1  "<True Position Y>"
  Bus Selector/3 -> Simulink-PS Converter2/1  "<True Orientation>"
  True Position States/1 -> Bus Selector/1
  connections:
  Vehicle Base Chasis/RConn1 -- Left Wheel/LConn1 -- Right Wheel/LConn1 -- Rigid Transform/RConn1
  Simulink-PS Converter1/RConn1 -- Planar Joint/LConn3
  Simulink-PS Converter2/RConn1 -- Planar Joint/LConn4
  World Link/RConn1 -- Planar Joint/LConn1
  Simulink-PS Converter/RConn1 -- Planar Joint/LConn2
  Rigid Transform/LConn1 -- Planar Joint/RConn1

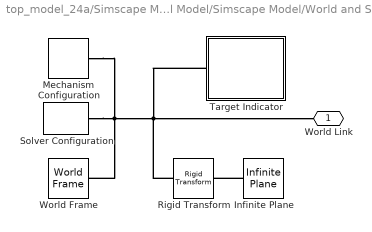
== system top_model_24a/Simscape Multibody Physical Model/Simscape Model/World and Solver ==
  Infinite Plane : sm_lib/Curves and Surfaces/Infinite Plane  GraphicType=Rectangle  GraphicPlaneWidth=world.plane.dimentionX  GraphicPlaneWidthUnits=m  GraphicPlaneHeight=world.plane.dimentionY  GraphicPlaneHeightUnits=m  GraphicVisPropType=SimpleVisualProperties  GraphicDiffuseColor=world.plane.colour  GraphicOpacity=world.plane.opacity  GraphicSpecularColor=[0.5 0.5 0.5 1.0]  GraphicAmbientColor=[0.15 0.15 0.15 1.0]  GraphicEmissiveColor=[0.0 0.0 0.0 1.0]  GraphicShininess=75
  Mechanism Configuration : sm_lib/Utilities/Mechanism Configuration  UniformGravity=Constant  GravityVector=[0 0 0]  GravityVectorUnits=m/s^2  LinearizationDelta=0.001  JointModeTransitionNonlinearIterations=2
  Rigid Transform : sm_lib/Frames and Transforms/Rigid Transform  RotationMethod=None  FollAlignAxisA=+X  BaseAlignAxisA=+Y  FollAlignAxisB=+Y  BaseAlignAxisB=+Z  RotationStandardAxis=+Z  RotationAngle=0  RotationAngleUnits=deg  RotationArbitraryAxis=[0 0 1]  RotationSequenceAxes=FollowerAxes  RotationSequence=XYX  RotationSequenceAngles=[0 0 0]  RotationSequenceAnglesUnits=deg  RotationMatrix=[1 0 0;0 1 0;0 0 1]  Quaternion=[1 0 0 0]  TranslationMethod=StandardAxis  TranslationCartesianOffset=[0 0 0]  TranslationCartesianOffsetUnits=m  TranslationStandardAxis=-Z  TranslationStandardOffset=0  TranslationStandardOffsetUnits=m  TranslationROffset=0  TranslationROffsetUnits=m  TranslationThetaOffset=0  TranslationThetaOffsetUnits=deg  TranslationZOffset=0  TranslationZOffsetUnits=m
  Solver Configuration : nesl_utility/Solver Configuration  PhysicalDomain=network_engine_domain  SubClassName=solver  LeftPortType=input  RightPortType=generic  Tones=[]  Harmonics=[]  SimulateNoise=off  Profile=off  UseLocalSampling=off  EnableSwitchedLinearOptims=on  FrequencyDomain=off  UseCCode=off  RelTol=0.001  AbsTol=0.001  MinStep=1e-09  ToWorkspace=off  RevertToSquareIcSolve=off  NumHomotopyIterations=100  PhasorMode=off  PhasorModeNumHarmonics=1  ConsistencySolver=NEWTON_XTOL_AFTER_FTOL  IndexReductionMethod=DerivativeReplacement  DoDC=off  ResidualTolerance=1e-09  ConsistencyTolSource=GLOBAL  ConsistencyAbsTol=0.001  ConsistencyRelTol=0.001  ConsistencyTolFactor=0.001  UseLocalSolver=off  LocalSolverChoice=NE_BACKWARD_EULER_ADVANCER  ResolveIndetEquations=on  FunctionEvalNumThread=1  LocalSolverSampleTime=0.001  DoFixedCost=off  MaxNonlinIter=3  MaxModeIter=2  ComputeImpulses=off  ImpulseIterations=2  LinearAlgebra=auto  LinearAlgebraNumThread=0  EquationFormulation=NE_TIME_EF  DelaysMemoryBudget=1024  AutomaticFiltering=on  FilteringTimeConstant=0.001  PartitionStorageMethod=AS_NEEDED  PartitionMemoryBudget=1024  PartitionMethod=ROBUST  MultibodyUseLocalSolver=off  MultibodyLocalSolverChoice=ODE1  MultibodyLocalSolverSampleTime=0.001
  Target Indicator : Subsystem
  World Frame : sm_lib/Frames and Transforms/World Frame
  World Link : PMIOPort  Side=Right
  connections:
  Mechanism Configuration/RConn1 -- Target Indicator/LConn1 -- Rigid Transform/LConn1 -- World Link/RConn1 -- Solver Configuration/RConn1 -- World Frame/RConn1
  Infinite Plane/LConn1 -- Rigid Transform/RConn1

== system top_model_24a/Simscape Multibody Physical Model/Simscape Model/Vehicle Base/Left Wheel ==
  Left Wheel : sm_lib/Body Elements/Cylindrical Solid  CylinderRadius=vehicle.wheel.radius  CylinderRadiusUnits=m  CylinderLength=vehicle.wheel.width  CylinderLengthUnits=m  ExportEntireGeometry=off  InertiaType=CalculateFromGeometry  BasedOnType=Mass  Density=1000  DensityUnits=kg/m^3  Mass=vehicle.wheel.mass  MassUnits=kg  CenterOfMass=[0 0 0]  CenterOfMassUnits=m  MomentsOfInertia=[1 1 1]  MomentsOfInertiaUnits=kg*m^2  ProductsOfInertia=[0 0 0]  ProductsOfInertiaUnits=kg*m^2  GraphicType=FromGeometry  MarkerShape=Sphere  MarkerSize=10  GraphicVisPropType=SimpleVisualProperties  GraphicDiffuseColor=vehicle.wheel.colour  GraphicOpacity=vehicle.wheel.opacity  GraphicSpecularColor=[0.5 0.5 0.5 1.0]  GraphicAmbientColor=[0.15 0.15 0.15 1.0]  GraphicEmissiveColor=[0.0 0.0 0.0 1.0]  GraphicShininess=75  DoExposeReferenceFrame=on  SerializedFrames=<Frames/>
  Rigid Transform1 : sm_lib/Frames and Transforms/Rigid Transform  RotationMethod=StandardAxis  FollAlignAxisA=+X  BaseAlignAxisA=+Y  FollAlignAxisB=+Y  BaseAlignAxisB=+Z  RotationStandardAxis=+X  RotationAngle=90  RotationAngleUnits=deg  RotationArbitraryAxis=[0 0 1]  RotationSequenceAxes=FollowerAxes  RotationSequence=XYX  RotationSequenceAngles=[0 0 0]  RotationSequenceAnglesUnits=deg  RotationMatrix=[1 0 0;0 1 0;0 0 1]  Quaternion=[1 0 0 0]  TranslationMethod=StandardAxis  TranslationCartesianOffset=[0 0 0]  TranslationCartesianOffsetUnits=m  TranslationStandardAxis=+Y  TranslationStandardOffset=vehicle.trackWidth/2  TranslationStandardOffsetUnits=m  TranslationROffset=0  TranslationROffsetUnits=m  TranslationThetaOffset=0  TranslationThetaOffsetUnits=deg  TranslationZOffset=0  TranslationZOffsetUnits=m
  Conn1 : PMIOPort  Side=Left
  connections:
  Rigid Transform1/LConn1 -- Conn1/RConn1
  Rigid Transform1/RConn1 -- Left Wheel/RConn1

== system top_model_24a/Simscape Multibody Physical Model/Simscape Model/Vehicle Base/Right Wheel ==
  Right Wheel : sm_lib/Body Elements/Cylindrical Solid  CylinderRadius=vehicle.wheel.radius  CylinderRadiusUnits=m  CylinderLength=vehicle.wheel.width  CylinderLengthUnits=m  ExportEntireGeometry=off  InertiaType=CalculateFromGeometry  BasedOnType=Mass  Density=1000  DensityUnits=kg/m^3  Mass=vehicle.wheel.mass  MassUnits=kg  CenterOfMass=[0 0 0]  CenterOfMassUnits=m  MomentsOfInertia=[1 1 1]  MomentsOfInertiaUnits=kg*m^2  ProductsOfInertia=[0 0 0]  ProductsOfInertiaUnits=kg*m^2  GraphicType=FromGeometry  MarkerShape=Sphere  MarkerSize=10  GraphicVisPropType=SimpleVisualProperties  GraphicDiffuseColor=vehicle.wheel.colour  GraphicOpacity=vehicle.wheel.opacity  GraphicSpecularColor=[0.5 0.5 0.5 1.0]  GraphicAmbientColor=[0.15 0.15 0.15 1.0]  GraphicEmissiveColor=[0.0 0.0 0.0 1.0]  GraphicShininess=75  DoExposeReferenceFrame=on  SerializedFrames=<Frames/>
  Rigid Transform2 : sm_lib/Frames and Transforms/Rigid Transform  RotationMethod=StandardAxis  FollAlignAxisA=+X  BaseAlignAxisA=+Y  FollAlignAxisB=+Y  BaseAlignAxisB=+Z  RotationStandardAxis=+X  RotationAngle=-90  RotationAngleUnits=deg  RotationArbitraryAxis=[0 0 1]  RotationSequenceAxes=FollowerAxes  RotationSequence=XYX  RotationSequenceAngles=[0 0 0]  RotationSequenceAnglesUnits=deg  RotationMatrix=[1 0 0;0 1 0;0 0 1]  Quaternion=[1 0 0 0]  TranslationMethod=StandardAxis  TranslationCartesianOffset=[0 0 0]  TranslationCartesianOffsetUnits=m  TranslationStandardAxis=-Y  TranslationStandardOffset=vehicle.trackWidth/2  TranslationStandardOffsetUnits=m  TranslationROffset=0  TranslationROffsetUnits=m  TranslationThetaOffset=0  TranslationThetaOffsetUnits=deg  TranslationZOffset=0  TranslationZOffsetUnits=m
  Conn1 : PMIOPort  Side=Left
  connections:
  Rigid Transform2/LConn1 -- Conn1/RConn1
  Rigid Transform2/RConn1 -- Right Wheel/RConn1

== system top_model_24a/Simscape Multibody Physical Model/Simscape Model/World and Solver/Target Indicator ==
  Demux : Demux  Outputs=2
  Rectangular Joint : sm_lib/Joints/Rectangular Joint  JointMode=Normal  CompositeWrenchDir=FollowerOnBase  CompositeWrenchFrame=BaseFrame  SenseConstraintForce=off  SenseConstraintTorque=off  SenseTotalForce=off  SenseTotalTorque=off  PxPositionTargetSpecify=off  PxPositionTargetPriority=High  PxPositionTargetValue=0  PxPositionTargetValueUnits=m  PxVelocityTargetSpecify=off  PxVelocityTargetPriority=High  PxVelocityTargetValue=0  PxVelocityTargetValueUnits=m/s  PxEquilibriumPosition=0  PxEquilibriumPositionUnits=m  PxSpringStiffness=0  PxSpringStiffnessUnits=N/m  PxDampingCoefficient=0  PxDampingCoefficientUnits=N/(m/s)  PxLowerLimitSpecify=off  PxLowerLimitBound=-1  PxLowerLimitBoundUnits=m  PxLowerLimitStiffness=1e6  PxLowerLimitStiffnessUnits=N/m  PxLowerLimitDamping=1e3  PxLowerLimitDampingUnits=N/(m/s)  PxLowerLimitTransitionRegionWidth=1e-4  PxLowerLimitTransitionRegionWidthUnits=m  PxUpperLimitSpecify=off  PxUpperLimitBound=1  PxUpperLimitBoundUnits=m  PxUpperLimitStiffness=1e6  PxUpperLimitStiffnessUnits=N/m  PxUpperLimitDamping=1e3  PxUpperLimitDampingUnits=N/(m/s)  PxUpperLimitTransitionRegionWidth=1e-4  PxUpperLimitTransitionRegionWidthUnits=m  PxTorqueActuationMode=ComputedTorque  PxMotionActuationMode=InputMotion  PxSensePosition=off  PxSenseVelocity=off  PxSenseAcceleration=off  PxSenseTorqueForce=off  PxSenseLowerLimitTorqueForce=off  PxSenseUpperLimitTorqueForce=off  PyPositionTargetSpecify=off  PyPositionTargetPriority=High  PyPositionTargetValue=0  PyPositionTargetValueUnits=m  PyVelocityTargetSpecify=off  PyVelocityTargetPriority=High  PyVelocityTargetValue=0  PyVelocityTargetValueUnits=m/s  PyEquilibriumPosition=0  PyEquilibriumPositionUnits=m  PySpringStiffness=0  PySpringStiffnessUnits=N/m  PyDampingCoefficient=0  PyDampingCoefficientUnits=N/(m/s)  PyLowerLimitSpecify=off  PyLowerLimitBound=-1  PyLowerLimitBoundUnits=m  PyLowerLimitStiffness=1e6  PyLowerLimitStiffnessUnits=N/m  PyLowerLimitDamping=1e3  PyLowerLimitDampingUnits=N/(m/s)  PyLowerLimitTransitionRegionWidth=1e-4  PyLowerLimitTransitionRegionWidthUnits=m  PyUpperLimitSpecify=off  PyUpperLimitBound=1  PyUpperLimitBoundUnits=m  PyUpperLimitStiffness=1e6  PyUpperLimitStiffnessUnits=N/m  PyUpperLimitDamping=1e3  PyUpperLimitDampingUnits=N/(m/s)  PyUpperLimitTransitionRegionWidth=1e-4  PyUpperLimitTransitionRegionWidthUnits=m  PyTorqueActuationMode=ComputedTorque  PyMotionActuationMode=InputMotion  PySensePosition=off  PySenseVelocity=off  PySenseAcceleration=off  PySenseTorqueForce=off  PySenseLowerLimitTorqueForce=off  PySenseUpperLimitTorqueForce=off
  Simulink-PS Converter3 : nesl_utility/Simulink-PS Converter  PhysicalDomain=network_engine_domain  SubClassName=ps_input  LeftPortType=input  RightPortType=output  PseudoPeriodic=off  Frequencies=[]  NoiseDistribution=none  NoiseParameters=[]  Unit=1  AffineConversion=off  FilteringAndDerivatives=filter  SimscapeFilterOrder=2  InputFilterTimeConstant=0.001  UdotUserProvided=0
  Simulink-PS Converter4 : nesl_utility/Simulink-PS Converter  PhysicalDomain=network_engine_domain  SubClassName=ps_input  LeftPortType=input  RightPortType=output  PseudoPeriodic=off  Frequencies=[]  NoiseDistribution=none  NoiseParameters=[]  Unit=1  AffineConversion=off  FilteringAndDerivatives=filter  SimscapeFilterOrder=2  InputFilterTimeConstant=0.001  UdotUserProvided=0
  Spherical Solid : sm_lib/Body Elements/Spherical Solid  SphereRadius=target.radius  SphereRadiusUnits=m  ExportEntireGeometry=off  InertiaType=CalculateFromGeometry  BasedOnType=Mass  Density=1000  DensityUnits=kg/m^3  Mass=0  MassUnits=kg  CenterOfMass=[0 0 0]  CenterOfMassUnits=m  MomentsOfInertia=[1 1 1]  MomentsOfInertiaUnits=kg*m^2  ProductsOfInertia=[0 0 0]  ProductsOfInertiaUnits=kg*m^2  GraphicType=FromGeometry  MarkerShape=Sphere  MarkerSize=10  GraphicVisPropType=SimpleVisualProperties  GraphicDiffuseColor=target.colour  GraphicOpacity=target.opacity  GraphicSpecularColor=[0.5 0.5 0.5 1.0]  GraphicAmbientColor=[0.15 0.15 0.15 1.0]  GraphicEmissiveColor=[0.0 0.0 0.0 1.0]  GraphicShininess=75  DoExposeReferenceFrame=on  SerializedFrames=<Frames/>
  Conn1 : PMIOPort  Side=Left
  wires:
  Demux/2 -> Simulink-PS Converter4/1
  Demux/1 -> Simulink-PS Converter3/1
  [waypoint] -> Demux/1
  connections:
  Simulink-PS Converter4/RConn1 -- Rectangular Joint/LConn3
  Rectangular Joint/RConn1 -- Spherical Solid/RConn1
  Simulink-PS Converter3/RConn1 -- Rectangular Joint/LConn2
  Rectangular Joint/LConn1 -- Conn1/RConn1

== matlab function top_model_24a/Control System/Control Logic/PID Controllers/MATLAB Function ==
  data: heading_error input; heading_error_wrapped output
function heading_error_wrapped = fcn(heading_error)

heading_error_wrapped = atan2(sin(heading_error), cos(heading_error));

== matlab function top_model_24a/Motion Planning & Reference Generation (Waypoints)/MATLAB Function ==
  data: t input; position_X output; maxLinearVelocity input; position_Y output
function [position_X, position_Y] = figureEightPath(t, maxLinearVelocity)
% Generate (x, y) for a vehicle on a figure-eight path at time t

% === Parameters ===
A = 8;  % Horizontal size of the figure eight
B = 8;  % Vertical size (half of A for symmetry)

% Estimate a base angular frequency based on desired velocity
% This assumes a typical path length of approx 2A + 2B
approx_path_length = 2*A + 2*B;
T = approx_path_length / (maxLinearVelocity/3); % estimated period
omega = 2*pi / T;

% === Figure-Eight Path (Lissajous curve) ===
x = A * sin(omega * t);
y = B * sin(2 * omega * t);

position_X = x;
position_Y = y;

end

== matlab function top_model_24a/Motion Planning & Reference Generation (Waypoints)/MATLAB Function1 ==
  data: t input; position_X output; maxLinearVelocity input; position_Y output
function [position_X, position_Y]  = circularPath(t, maxLinearVelocity)
% Generate (x, y) for a vehicle on a circular path at time t

% ==== Parameters ====
r = 8;              % Radius of the circle [m]
omega = maxLinearVelocity/r;          % Angular speed [rad/s]

% ==== Circular Path ====
theta = omega * t;    % Angle at time t
x = r * cos(theta);
y = r * sin(theta);

position_X = x;
position_Y = y;

== matlab function top_model_24a/Sensor Model/Sensors/Camera/MATLAB Function ==
  data: pose input; I output
function I = fakeCamera(pose)
% pose is [x; y; theta]
% I must be a H×W×3 uint8 image for Video Viewer.

% Example placeholder: draw a colored circle whose position depends on pose
H = 224; W = 224;
I = zeros(H, W, 3, 'uint8');

% Map world x,y into pixel:
u = round( (pose(1)+5) / 10 * (W-1) ) + 1;
v = round( (pose(2)+5) / 10 * (H-1) ) + 1;
u = min(max(u,1),W);
v = min(max(v,1),H);

% Draw a small red dot:
radius = 5;
[xx,yy] = meshgrid(1:W,1:H);
mask = (xx-u).^2 + (yy-v).^2 <= radius^2;
I(:,:,1) = uint8(mask) * 255; % red channel

end

== matlab function top_model_24a/Visual Sensor Model/MATLAB Function ==
  data: dx output; dy output; distance output; target_angle output; heading_error output; vehiclePose input; objectPos input; I output; ballRadius input; ballColor input
function [dx, dy, distance, target_angle, heading_error, I] = fakeCameraPOV(vehiclePose, objectPos, ballRadius, ballColor)
% Simulate a camera image from the vehicle's point of view, indicating if the target is in FOV.
% Inputs:
%   vehiclePose: [x_v; y_v; theta_v] - vehicle's world position (x_v, y_v) and heading (theta_v in radians)
%   objectPos: [x_o; y_o] - object's world position from figureEightPath
%   ballRadius: scalar - radius of the ball in world units (unused)
%   ballColor: 1×3 vector [R G B] - color of the ball
% Output:
%   I: H×W×3 uint8 image for Simulink Video Viewer (target color if in FOV, black if not)

% Image dimensions
H = 224; W = 224;
I = zeros(H, W, 3, 'uint8'); % Initialize black image

% Camera parameters
max_distance = 20; % Maximum viewable distance (matches world size)
fov = deg2rad(120); % Field of view (120 degrees)

% Extract inputs
x_v = vehiclePose(1); y_v = vehiclePose(2); theta_v = vehiclePose(3);
x_o = objectPos(1); y_o = objectPos(2);

% Compute direct distance in world frame
dx = x_o - x_v;
dy = y_o - y_v;
% dx = x_v - x_o;
% dy = y_v - y_o;
distance = sqrt(dx^2 + dy^2);

% Compute angle to target in world frame
target_angle = atan2(dy, dx); % Angle of target relative to positive x-axis

% Compute heading error (difference between robot heading and target angle)
heading_error = target_angle - theta_v;
heading_error = mod(heading_error + pi, 2*pi) - pi; % Normalize to [-pi, pi]

% Check if object is within range and FOV
if distance <= max_distance && abs(heading_error) <= fov/2
    % Target is in FOV: set image to target color
    I(:,:,1) = ballColor(1); % Red channel
    I(:,:,2) = ballColor(2); % Green channel
    I(:,:,3) = ballColor(3); % Blue channel
else
    % Target not in FOV: leave image black
    I = I; % Already black
end

end
